simulink model "statefeedbacknonlin"  (R2019b)
settings: Solver=VariableStepAuto  StartTime=0.0  StopTime=10.0  RelTol=1e-3
values from neighbouring files (symbols this model uses):
  A = [-1/9 1/9;1/9 -0.3889]    [lqrfeedback_params.m]    (also in observerbasednonlin_params.m = 0.01; observerdesign_params.m; statefeedback_params.m; statefeedbacknonlin_params.m = 0.01)
  g = 9.81    [observerbasednonlin_params.m]    (also in statefeedbacknonlin_params.m)
  h1eq = 0    [lqrfeedback_params.m]    (also in observerbasednonlin_params.m; observerdesign_params.m; statefeedback_params.m; statefeedbacknonlin_params.m)
  h1init = 0    [statefeedback_params.m]    (also in statefeedbacknonlin_params.m = 0.05)
  h2eq = 0    [lqrfeedback_params.m]    (also in observerbasednonlin_params.m; observerdesign_params.m; statefeedback_params.m; statefeedbacknonlin_params.m)
  h2init = 1    [statefeedback_params.m]    (also in statefeedbacknonlin_params.m = 0.03)
  k1 = k(1)    [lqrfeedback_params.m]    (also in observerbasednonlin_params.m = 1.095; observerdesign_params.m = 0.0151; statefeedback_params.m = 1.09; statefeedbacknonlin_params.m = 1.09)
  k2 = k(2)    [lqrfeedback_params.m]    (also in observerbasednonlin_params.m = 87.12; observerdesign_params.m = 0.3997; statefeedback_params.m = 86.1515; statefeedbacknonlin_params.m = 86.1515)
  ro = 1    [observerbasednonlin_params.m]    (also in statefeedbacknonlin_params.m)
  ro1 = 1.262*10e-4    (= 0.001262)    [observerbasednonlin_params.m]    (also in statefeedbacknonlin_params.m = 178.57)
  ro2 = 1.262*10e-4    (= 0.001262)    [observerbasednonlin_params.m]    (also in statefeedbacknonlin_params.m = 178.57)
settings Model: Creator=SAI JOSHITHA  LastModifiedBy=SAI JOSHITHA

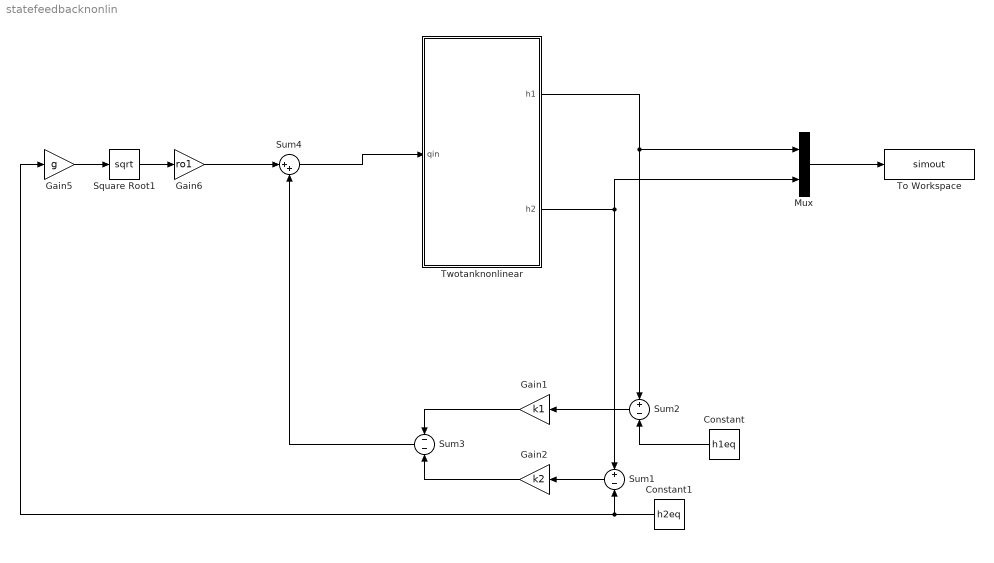
== system statefeedbacknonlin ==
  Constant : Constant  Value=h1eq
  Constant1 : Constant  Value=h2eq
  Gain1 : Gain  Gain=k1
  Gain2 : Gain  Gain=k2
  Gain5 : Gain  Gain=g
  Gain6 : Gain  Gain=ro1
  Mux : Mux  Inputs=2
  Square Root1 : Sqrt  SaturateOnIntegerOverflow=on
  Sum1 : Sum  Inputs=+-
  Sum2 : Sum  Inputs=+-
  Sum3 : Sum  Inputs=--
  Sum4 : Sum  Inputs=|++
  To Workspace : ToWorkspace  VariableName=simout  SaveFormat=Timeseries  SampleTime=-1
  Twotanknonlinear : Subsystem
  wires:
  Sum2/1 -> Gain1/1
  Gain1/1 -> Sum3/1
  Gain2/1 -> Sum3/2
  Constant/1 -> Sum2/2
  Sum1/1 -> Gain2/1
  Sum4/1 -> Twotanknonlinear/1(qin)
  Sum3/1 -> Sum4/2
  Mux/1 -> To Workspace/1
  Constant1/1 -> Gain5/1, Sum1/2
  Twotanknonlinear/1(h1) -> Mux/1, Sum2/1
  Twotanknonlinear/2(h2) -> Sum1/1, Mux/2
  Gain5/1 -> Square Root1/1
  Square Root1/1 -> Gain6/1
  Gain6/1 -> Sum4/1

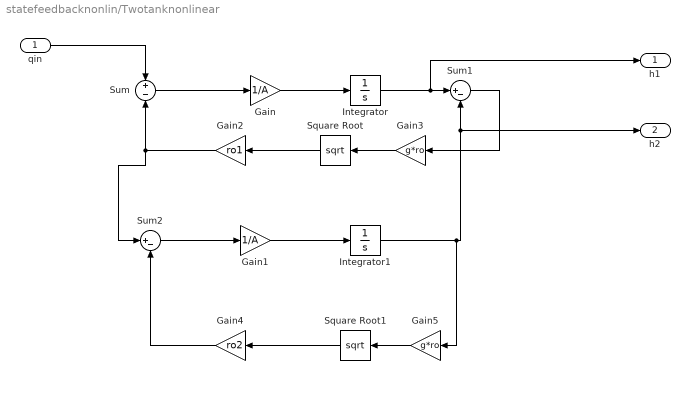
== system statefeedbacknonlin/Twotanknonlinear ==
  qin : Inport
  Gain : Gain  Gain=1/A
  Gain1 : Gain  Gain=1/A
  Gain2 : Gain  Gain=ro1
  Gain3 : Gain  Gain=g*ro
  Gain4 : Gain  Gain=ro2
  Gain5 : Gain  Gain=g*ro
  Integrator : Integrator  InitialCondition=h1init
  Integrator1 : Integrator  InitialCondition=h2init
  Square Root : Sqrt  SaturateOnIntegerOverflow=on
  Square Root1 : Sqrt  SaturateOnIntegerOverflow=on
  Sum : Sum  Inputs=+-
  Sum1 : Sum  Inputs=|+-
  Sum2 : Sum  Inputs=|+-
  h1 : Outport
  h2 : Outport  Port=2
  wires:
  Gain3/1 -> Square Root/1
  Integrator/1 -> h1/1, Sum1/1
  Gain2/1 -> Sum2/1, Sum/2
  Sum2/1 -> Gain1/1
  Gain1/1 -> Integrator1/1
  Gain/1 -> Integrator/1
  Square Root/1 -> Gain2/1
  Sum/1 -> Gain/1
  Integrator1/1 -> Gain5/1, h2/1, Sum1/2
  Sum1/1 -> Gain3/1
  Square Root1/1 -> Gain4/1
  Gain5/1 -> Square Root1/1
  Gain4/1 -> Sum2/2
  qin/1 -> Sum/1
